simulink model "bpsk_mod"  (Simulink 7.2)
settings: Solver=ode45  StartTime=0.0  StopTime=0.02  RelTol=1e-3
undefined symbols (not defined in the file or in its folder): Fs, get
libraries: dspsnks4 x2
settings Model: Creator=Administrator  LastModifiedBy=Administrator
settings OptimizationCC: InitFltsAndDblsToZero=on

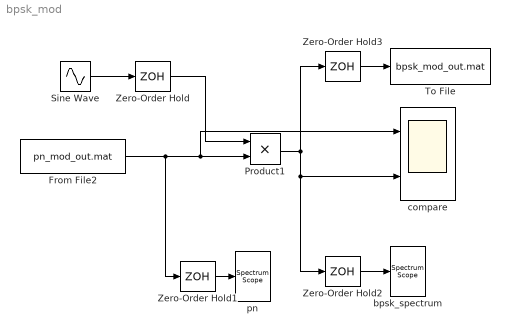
== system bpsk_mod ==
  From File2 : FromFile  FileName=pn_mod_out.mat  SampleTime=1/2.55e6
  Product1 : Product  OutDataType=sfix(16)  OutScaling=2^0  RndMeth=Zero
  Sine Wave : Sin  Frequency=510000*2*pi  SampleTime=1/10.2e6
  To File : ToFile  Filename=bpsk_mod_out.mat
  Zero-Order Hold{,1..3} (4 alike) : ZeroOrderHold  SampleTime=1/5.1e6
  bpsk_spectrum : dspsnks4/Spectrum Scope  DialogController=dspdialog.SpectrumScope  DialogControllerArgs=DataTag0  SystemSampleTime=-1  ScopeProperties=on  Domain=Frequency  HorizSpan=1  UseBuffer=on  BufferSize=512  Overlap=256  inpFftLenInherit=off  FFTlength=128  numAvg=2  DisplayProperties=off  AxisGrid=on  Memory=off  FrameNumber=on  AxisLegend=off  AxisZoom=off  OpenScopeAtSimStart=on  OpenScopeImmediately=off  FigPos=get(0,'defaultfigureposition')  AxisProperties=off  XUnits=Hertz  XRange=[-Fs/2...Fs/2]  XDisplay=0  InheritXIncr=on  XIncr=1.0  XLabel=Samples  XLimit=Auto  YUnits=dB  XMax=1  XMin=0  YLabel=Magnitude-squared, dB  LineProperties=off  wintypeSpecScope=Hann  RsSpecScope=50  betaSpecScope=5  winsampSpecScope=Periodic
      settings: YMin=-40.4645970991157  YMax=7.19960642620942
  compare : Scope  NumInputPorts=2
      settings: YMin=-1.5~-5  YMax=1.5~5
  pn : dspsnks4/Spectrum Scope  DialogController=dspdialog.SpectrumScope  DialogControllerArgs=DataTag1  SystemSampleTime=-1  ScopeProperties=on  Domain=Frequency  HorizSpan=1  UseBuffer=on  BufferSize=512  Overlap=256  inpFftLenInherit=off  FFTlength=128  numAvg=2  DisplayProperties=off  AxisGrid=on  Memory=off  FrameNumber=on  AxisLegend=off  AxisZoom=off  OpenScopeAtSimStart=on  OpenScopeImmediately=off  FigPos=get(0,'defaultfigureposition')  AxisProperties=off  XUnits=Hertz  XRange=[-Fs/2...Fs/2]  XDisplay=0  InheritXIncr=on  XIncr=1.0  XLabel=Samples  XLimit=Auto  YUnits=dB  XMax=1  XMin=0  YLabel=Magnitude-squared, dB  LineProperties=off  wintypeSpecScope=Hann  RsSpecScope=50  betaSpecScope=5  winsampSpecScope=Periodic
      settings: YMin=-47.6015123951546  YMax=20.0079847363653
  wires:
  Sine Wave/1 -> Zero-Order Hold/1
  Zero-Order Hold/1 -> Product1/1
  From File2/1 -> Zero-Order Hold1/1, Product1/2, compare/1
  Product1/1 -> Zero-Order Hold3/1, Zero-Order Hold2/1, compare/2
  Zero-Order Hold1/1 -> pn/1
  Zero-Order Hold2/1 -> bpsk_spectrum/1
  Zero-Order Hold3/1 -> To File/1
